simulink model "kinematics"  (R2015a)
settings: Solver=ode45  StartTime=0.0  StopTime=1000  RelTol=1e-3
settings Model: Creator=MCLab  LastModifiedBy=MCLab

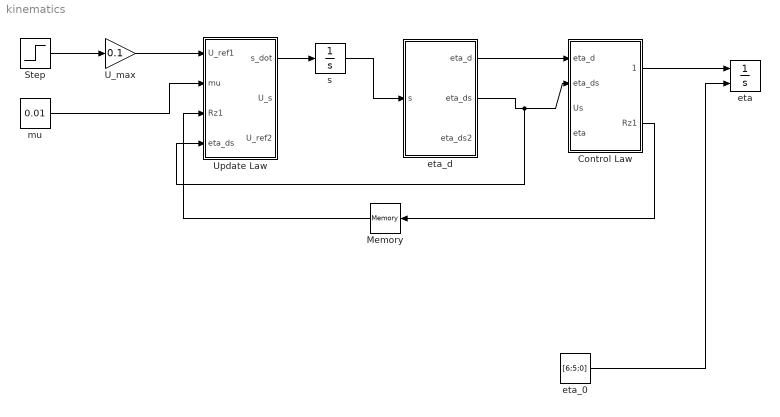
== system kinematics ==
  Control Law : MATLAB Function  TreatAsAtomicUnit=on
  Memory : Memory  X0=[0;0;0]
  Step : Step  Time=500  Before=1  After=-1  SampleTime=0
  U_max : Gain  Gain=0.1
  Update Law : MATLAB Function  TreatAsAtomicUnit=on
  eta : Integrator  InitialConditionSource=external
  eta_0 : Constant  Value=[6;5;0]
  eta_d : MATLAB Function  TreatAsAtomicUnit=on
  mu : Constant  Value=0.01
  s : Integrator
  wires:
  Step/1 -> U_max/1
  U_max/1 -> Update Law/1(U_ref1)
  mu/1 -> Update Law/2(mu)
  Update Law/1(s_dot) -> s/1
  s/1 -> eta_d/1(s)
  eta_d/1(eta_d) -> Control Law/1(eta_d)
  eta_d/2(eta_ds) -> Update Law/4(eta_ds), Control Law/2(eta_ds)
  Control Law/1(eta_dot) -> eta/1
  eta_0/1 -> eta/2
  Control Law/2(Rz1) -> Memory/1
  Memory/1 -> Update Law/3(Rz1)

== matlab function kinematics/eta_d ==
  data: s input; eta_d output; eta_ds output; eta_ds2 output
function [eta_d,eta_ds,eta_ds2] = fcn(s)

eta_d = [0;0;0];
eta_ds = [0;0;0];

% Straight Line

p_d0 = [2;0];
p_d1 = [10;4];

p_ds = [8;4];
p_d = p_d0 + s * p_ds ;

eta_d = [p_d;atan2(4,8)] ;
eta_ds = [p_ds;0];
eta_ds2 = [0;0;0];

end

== matlab function kinematics/Update Law ==
  data: U_ref1 input; s_dot output; mu input; Rz1 input; eta_ds input; U_s output; U_ref2 output
function [s_dot,U_s,U_ref2] = f(U_ref1,mu,Rz1,eta_ds)

% Straight Line

U_ref2 = U_ref1 ;

U_s = U_ref1 / sqrt(12^2+4^2);

V1 = - eta_ds'*Rz1 ;

s_dot = U_s - mu*V1/norm(eta_ds);

end

== matlab function kinematics/Control Law ==
  data: eta_d input; eta_ds input; Us input; eta input; eta_dot output; Rz1 output
function [eta_dot,Rz1] = fcn(eta_d,eta_ds,Us,eta)

psi = atan2(4,8);
eta_dot = [0;0;0];
nu = [0;0;0];

R = [ cos(psi) , -sin(psi) , 0 ;
      sin(psi) , cos(psi)  , 0 ;
      0            0         1 ] ;

K_p = diag([0.2,0.2,0.1]);

z1 = R'*(eta-eta_d);

Rz1 = R*z1 ;

alpha1 = -K_p*z1 + R'eta_ds*Us ;

nu = alpha1 ;

eta_dot = R*nu ;

end;
